simulink model "CompressorTest"  (R2019a)
settings: Solver=VariableStepAuto  StartTime=0.0  StopTime=604800  RelTol=1e-3
values from neighbouring files (symbols this model uses):
  lineParm = [lineParm;add_line("Main 3",24,35,pNom)]    [compressorTest.m]    (also in experiment1.m = [lineParm;add_line("Main 2",24,50,pNom)]; experiment2.m; experiment3.m = [lineParm;add_line("Aux 3",36,100,pNom)]; experiments12.m = [lineParm;add_line("Main 2",24,35,pNom)])
  loadParm = [loadParm; add_load("PP2",pwr,pNom,pCut, stopTime)]    [compressorTest.m]    (also in experiment1.m; experiment2.m; experiment3.m = [loadParm; add_load("PP2",pwr,pNom,pCut,stopTime)]; experiments12.m)
  loadState = "on"    [ColoradoGasModel.m]    (also in compressorTest.m = 'on'; experiment1.m = 'on'; experiment2.m = 'on'; experiment3.m = 'on')
libraries: fl_lib x16, gasLibrary x9, nesl_utility x6
(part 2 of 2)

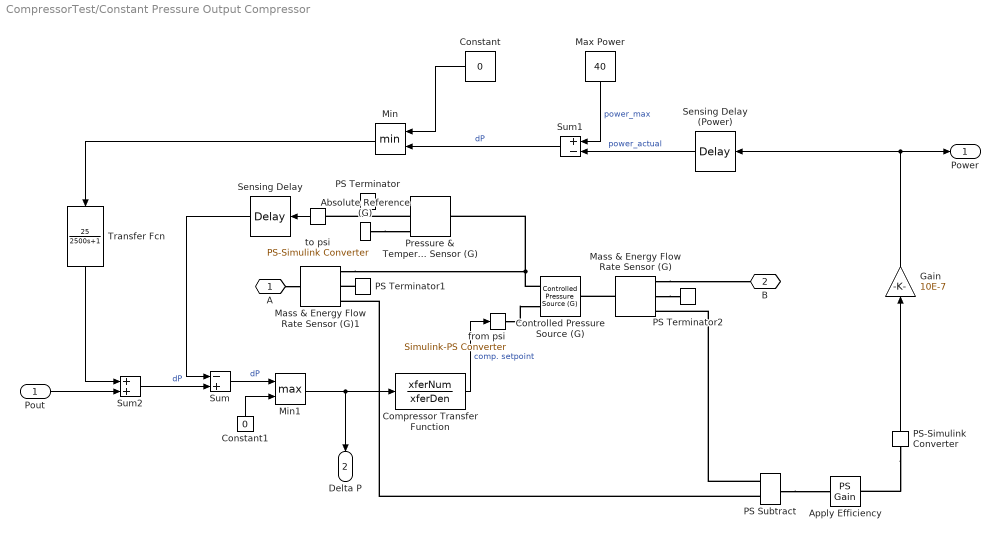
== system CompressorTest/Constant Pressure Output Compressor ==
  Pout : Inport
  Absolute Reference (G) : fl_lib/Gas/Elements/Absolute Reference (G)
      settings: SourceProductName=Simscape  SourceProductBaseCode=SS
  Apply Efficiency : fl_lib/Physical Signals/Functions/PS Gain  gain=1/efficiency
  Compressor Transfer Function : TransferFcn  Numerator=xferNum  Denominator=xferDen
  Constant : Constant  Value=0
  Constant1 : Constant  Value=0
  Controlled Pressure Source (G) : fl_lib/Gas/Sources/Controlled Pressure Source (G)  power_spec=1  area_A=24^2*pi/4 in^2  area_B=24^2*pi/4 in^2  mdot_A_specify=off  mdot_A_priority=None  mdot_A=1e-6 kg/s  mdot_A_nominal_specify=off  mdot_A_nominal_unit=kg/s  mdot_A_nominal_value=1
      settings: SourceProductName=Simscape  SourceProductBaseCode=SS
  Gain : Gain  Gain=10E-7
  Mass & Energy Flow Rate Sensor (G) : fl_lib/Gas/Sensors/Mass & Energy Flow Rate Sensor (G)
      settings: SourceProductName=Simscape  SourceProductBaseCode=SS
  Mass & Energy Flow Rate Sensor (G)1 : fl_lib/Gas/Sensors/Mass & Energy Flow Rate Sensor (G)
      settings: SourceProductName=Simscape  SourceProductBaseCode=SS
  Max Power : Constant  Value=40
  Min : MinMax  Inputs=2
  Min1 : MinMax  Function=max  Inputs=2
  PS Subtract : fl_lib/Physical Signals/Functions/PS Subtract
      settings: SourceProductName=Simscape
  PS Terminator : fl_lib/Physical Signals/Sinks/PS Terminator
      settings: SourceProductName=Simscape
  PS Terminator1 : fl_lib/Physical Signals/Sinks/PS Terminator
      settings: SourceProductName=Simscape
  PS Terminator2 : fl_lib/Physical Signals/Sinks/PS Terminator
      settings: SourceProductName=Simscape
  PS-Simulink Converter : nesl_utility/PS-Simulink Converter  PhysicalDomain=network_engine_domain  SubClassName=ps_output  LeftPortType=input  RightPortType=output  PseudoPeriodic=off  Frequencies=[]  Unit=W  AffineConversion=off
  Pressure & Temperature Sensor (G) : fl_lib/Gas/Sensors/Pressure & Temperature Sensor (G)
      settings: SourceProductName=Simscape  SourceProductBaseCode=SS
  Sensing Delay : TransportDelay  DelayTime=delaySeconds  TransDelayFeedthrough=on
  Sensing Delay (Power) : TransportDelay  DelayTime=delaySeconds  TransDelayFeedthrough=on
  Sum : Sum  Inputs=-+
  Sum1 : Sum  Inputs=+-
  Sum2 : Sum
  Transfer Fcn : TransferFcn  Numerator=[25]  Denominator=[2500 1]
  from psi : nesl_utility/Simulink-PS Converter  PhysicalDomain=network_engine_domain  SubClassName=ps_input  LeftPortType=input  RightPortType=output  PseudoPeriodic=off  Frequencies=[]  NoiseDistribution=none  NoiseParameters=[]  Unit=psi  AffineConversion=off  FilteringAndDerivatives=provide  SimscapeFilterOrder=1  InputFilterTimeConstant=0.001  UdotUserProvided=0
  to psi : nesl_utility/PS-Simulink Converter  PhysicalDomain=network_engine_domain  SubClassName=ps_output  LeftPortType=input  RightPortType=output  PseudoPeriodic=off  Frequencies=[]  Unit=psi  AffineConversion=off
  A : PMIOPort  Side=Left
  B : PMIOPort  Port=2  Side=Right
  Power : Outport
  Delta P : Outport  Port=2
  wires:
  Compressor Transfer Function/1 -> from psi/1  "comp. setpoint"
  Sensing Delay/1 -> Sum/1
  to psi/1 -> Sensing Delay/1
  Sensing Delay (Power)/1 -> Sum1/2  "power_actual"
  Max Power/1 -> Sum1/1  "power_max"
  Sum1/1 -> Min/2  "dP"
  Constant/1 -> Min/1
  Min/1 -> Transfer Fcn/1
  Pout/1 -> Sum2/2
  PS-Simulink Converter/1 -> Gain/1
  Gain/1 -> Power/1, Sensing Delay (Power)/1
  Sum2/1 -> Sum/2  "dP"
  Sum/1 -> Min1/1  "dP"
  Min1/1 -> Delta P/1, Compressor Transfer Function/1
  Constant1/1 -> Min1/2
  Transfer Fcn/1 -> Sum2/1
  connections:
  Absolute Reference (G)/LConn1 -- Pressure & Temperature Sensor (G)/RConn1
  Pressure & Temperature Sensor (G)/RConn2 -- to psi/LConn1
  from psi/RConn1 -- Controlled Pressure Source (G)/LConn2
  PS Terminator/LConn1 -- Pressure & Temperature Sensor (G)/RConn3
  Controlled Pressure Source (G)/LConn1 -- Mass & Energy Flow Rate Sensor (G)1/RConn1 -- Pressure & Temperature Sensor (G)/LConn1
  Mass & Energy Flow Rate Sensor (G)/LConn1 -- Controlled Pressure Source (G)/RConn1
  Mass & Energy Flow Rate Sensor (G)/RConn1 -- B/RConn1
  A/RConn1 -- Mass & Energy Flow Rate Sensor (G)1/LConn1
  PS Terminator1/LConn1 -- Mass & Energy Flow Rate Sensor (G)1/RConn2
  Mass & Energy Flow Rate Sensor (G)/RConn2 -- PS Terminator2/LConn1
  PS Subtract/LConn1 -- Mass & Energy Flow Rate Sensor (G)/RConn3
  PS Subtract/LConn2 -- Mass & Energy Flow Rate Sensor (G)1/RConn3
  PS Subtract/RConn1 -- Apply Efficiency/LConn1
  PS-Simulink Converter/LConn1 -- Apply Efficiency/RConn1

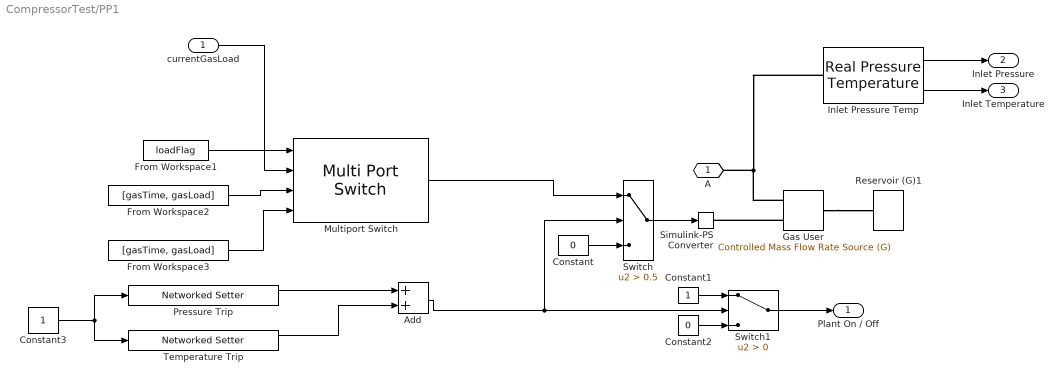
== system CompressorTest/PP1 ==
  currentGasLoad : Inport
  Add : Sum
  Constant : Constant  Value=0
  Constant1 : Constant
  Constant2 : Constant  Value=0
  Constant3 : Constant
  From Workspace1 : FromWorkspace  VariableName=loadFlag  SampleTime=0
  From Workspace2 : FromWorkspace  VariableName=[gasTime, gasLoad]  SampleTime=0
  From Workspace3 : FromWorkspace  VariableName=[gasTime, gasLoad]  SampleTime=0
  Gas User : fl_lib/Gas/Sources/Controlled Mass Flow Rate Source (G)  power_spec=1  area_A=24^2*pi/4 in^2  area_B=20^2*pi/4 in^2  mdot_A_specify=on  mdot_A_priority=None  mdot_A=20 kg/s  mdot_A_nominal_specify=off  mdot_A_nominal_unit=kg/s  mdot_A_nominal_value=1
      settings: SourceProductName=Simscape  SourceProductBaseCode=SS
  Inlet Pressure Temp : gasLibrary/Real Pressure Temperature  SystemSampleTime=-1
  Multiport Switch : MultiPortSwitch
  Pressure Trip : gasLibrary/Networked Setter  LocalPort=pressurePort
  Reservoir (G)1 : fl_lib/Gas/Elements/Reservoir (G)  pressure_spec=2  reservoir_pressure=300 psi  reservoir_temperature=25 degC  area_A=pi*25^2/4 in^2
      settings: SourceProductName=Foundation Library
  Simulink-PS Converter : nesl_utility/Simulink-PS Converter  PhysicalDomain=network_engine_domain  SubClassName=ps_input  LeftPortType=input  RightPortType=output  PseudoPeriodic=off  Frequencies=[]  NoiseDistribution=none  NoiseParameters=[]  Unit=1  AffineConversion=off  FilteringAndDerivatives=provide  SimscapeFilterOrder=1  InputFilterTimeConstant=0.001  UdotUserProvided=0
  Switch : Switch  Criteria=u2 > Threshold  Threshold=0.5
  Switch1 : Switch  Criteria=u2 > Threshold
  Temperature Trip : gasLibrary/Networked Setter  LocalPort=temperaturePort
  A : PMIOPort  Side=Left
  Plant On / Off : Outport
  Inlet Pressure : Outport  Port=2
  Inlet Temperature : Outport  Port=3
  wires:
  Inlet Pressure Temp/2 -> Inlet Temperature/1
  Inlet Pressure Temp/1 -> Inlet Pressure/1
  Constant1/1 -> Switch1/1
  Switch1/1 -> Plant On / Off/1
  Constant2/1 -> Switch1/3
  Switch/1 -> Simulink-PS Converter/1
  Constant/1 -> Switch/3
  Multiport Switch/1 -> Switch/1
  From Workspace1/1 -> Multiport Switch/1
  From Workspace2/1 -> Multiport Switch/3
  From Workspace3/1 -> Multiport Switch/4
  currentGasLoad/1 -> Multiport Switch/2
  Add/1 -> Switch/2, Switch1/2
  Temperature Trip/1 -> Add/2
  Pressure Trip/1 -> Add/1
  Constant3/1 -> Pressure Trip/1, Temperature Trip/1
  connections:
  Gas User/LConn2 -- Simulink-PS Converter/RConn1
  Inlet Pressure Temp/LConn1 -- A/RConn1 -- Gas User/LConn1
  Gas User/RConn1 -- Reservoir (G)1/LConn1

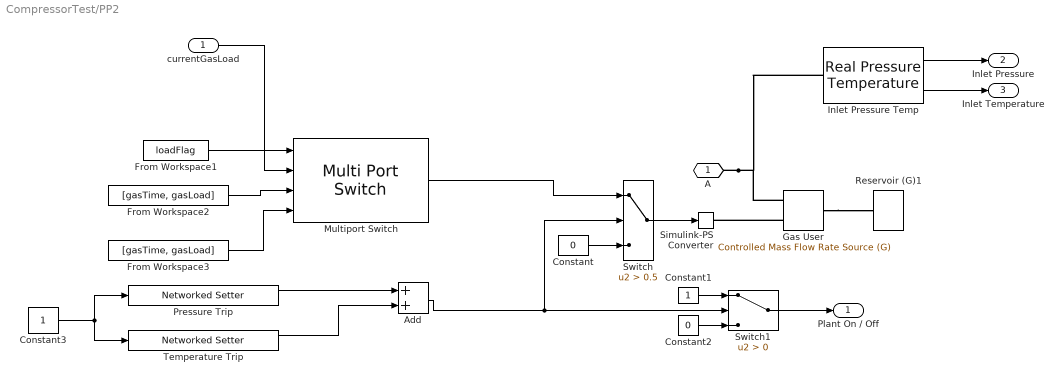
== system CompressorTest/PP2 ==
  currentGasLoad : Inport
  Add : Sum
  Constant : Constant  Value=0
  Constant1 : Constant
  Constant2 : Constant  Value=0
  Constant3 : Constant
  From Workspace1 : FromWorkspace  VariableName=loadFlag  SampleTime=0
  From Workspace2 : FromWorkspace  VariableName=[gasTime, gasLoad]  SampleTime=0
  From Workspace3 : FromWorkspace  VariableName=[gasTime, gasLoad]  SampleTime=0
  Gas User : fl_lib/Gas/Sources/Controlled Mass Flow Rate Source (G)  power_spec=1  area_A=24^2*pi/4 in^2  area_B=20^2*pi/4 in^2  mdot_A_specify=on  mdot_A_priority=None  mdot_A=20 kg/s  mdot_A_nominal_specify=off  mdot_A_nominal_unit=kg/s  mdot_A_nominal_value=1
      settings: SourceProductName=Simscape  SourceProductBaseCode=SS
  Inlet Pressure Temp : gasLibrary/Real Pressure Temperature  SystemSampleTime=-1
  Multiport Switch : MultiPortSwitch
  Pressure Trip : gasLibrary/Networked Setter  LocalPort=pressurePort
  Reservoir (G)1 : fl_lib/Gas/Elements/Reservoir (G)  pressure_spec=2  reservoir_pressure=300 psi  reservoir_temperature=25 degC  area_A=pi*25^2/4 in^2
      settings: SourceProductName=Foundation Library
  Simulink-PS Converter : nesl_utility/Simulink-PS Converter  PhysicalDomain=network_engine_domain  SubClassName=ps_input  LeftPortType=input  RightPortType=output  PseudoPeriodic=off  Frequencies=[]  NoiseDistribution=none  NoiseParameters=[]  Unit=1  AffineConversion=off  FilteringAndDerivatives=provide  SimscapeFilterOrder=1  InputFilterTimeConstant=0.001  UdotUserProvided=0
  Switch : Switch  Criteria=u2 > Threshold  Threshold=0.5
  Switch1 : Switch  Criteria=u2 > Threshold
  Temperature Trip : gasLibrary/Networked Setter  LocalPort=temperaturePort
  A : PMIOPort  Side=Left
  Plant On / Off : Outport
  Inlet Pressure : Outport  Port=2
  Inlet Temperature : Outport  Port=3
  wires:
  Inlet Pressure Temp/2 -> Inlet Temperature/1
  Inlet Pressure Temp/1 -> Inlet Pressure/1
  Constant1/1 -> Switch1/1
  Switch1/1 -> Plant On / Off/1
  Constant2/1 -> Switch1/3
  Switch/1 -> Simulink-PS Converter/1
  Constant/1 -> Switch/3
  Multiport Switch/1 -> Switch/1
  From Workspace1/1 -> Multiport Switch/1
  From Workspace2/1 -> Multiport Switch/3
  From Workspace3/1 -> Multiport Switch/4
  currentGasLoad/1 -> Multiport Switch/2
  Add/1 -> Switch/2, Switch1/2
  Temperature Trip/1 -> Add/2
  Pressure Trip/1 -> Add/1
  Constant3/1 -> Pressure Trip/1, Temperature Trip/1
  connections:
  Gas User/LConn2 -- Simulink-PS Converter/RConn1
  A/RConn1 -- Inlet Pressure Temp/LConn1 -- Gas User/LConn1
  Gas User/RConn1 -- Reservoir (G)1/LConn1

== matlab function CompressorTest/Load Distributor ==
  data: powerPlantStates input; powerStationLoads output; loadProfile input
function powerStationLoads = fcn(powerPlantStates, loadProfile)

powerPlantStates=powerPlantStates==1;
loadsUp=sum(powerPlantStates);
if loadsUp == 0
    loadDist=0;
else
    loadDist=loadProfile / loadsUp;
end

powerStationLoads=powerPlantStates.*loadDist;
